simulink model "E01"  (R2014a)
settings: Solver=ode45  StartTime=0.0  StopTime=10  RelTol=1e-3
libraries: cstblocks x3
settings Model: Creator=Davide  LastModifiedBy=Davide

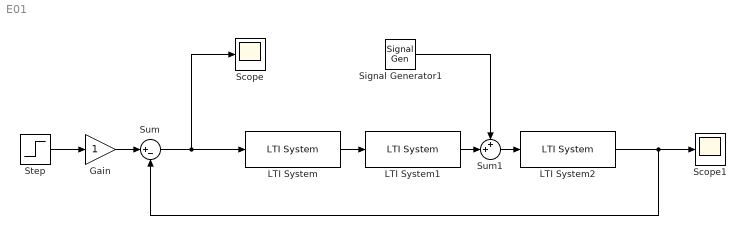
== system E01 ==
  Gain : Gain
  LTI System : cstblocks/LTI System  sys=Cz3  IC=[]
  LTI System1 : cstblocks/LTI System  sys=F1  IC=[]
  LTI System2 : cstblocks/LTI System  sys=F2  IC=[]
  Scope : Scope
  Scope1 : Scope
  Signal Generator1 : SignalGenerator  Amplitude=0  Frequency=200  Units=rad/sec
  Step : Step  Time=0  SampleTime=0
  Sum : Sum  Inputs=|+-
  Sum1 : Sum  Inputs=++|
  wires:
  LTI System/1 -> LTI System1/1
  Step/1 -> Gain/1
  Sum/1 -> Scope/1, LTI System/1
  LTI System2/1 -> Sum/2, Scope1/1
  Gain/1 -> Sum/1
  LTI System1/1 -> Sum1/2
  Sum1/1 -> LTI System2/1
  Signal Generator1/1 -> Sum1/1
